simulink model "Task1"  (R2016a)
settings: Solver=VariableStepAuto  StartTime=0.0  StopTime=10.0  RelTol=1e-3
settings Model: Creator=Thomas  LastModifiedBy=Thomas

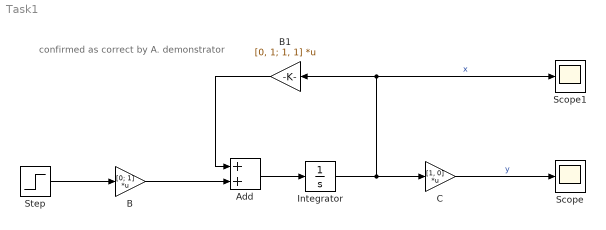
== system Task1 ==
  note: confirmed as correct by A. demonstrator
  Add : Sum
  B : Gain  Gain=[0; 1]  Multiplication=Matrix(K*u)
  B1 : Gain  Gain=[0, 1; 1, 1]  Multiplication=Matrix(K*u)
  C : Gain  Gain=[1, 0]  Multiplication=Matrix(K*u)
  Integrator : Integrator  InitialCondition=[1;1]
  Scope : Scope
  Scope1 : Scope
  Step : Step  SampleTime=0
  wires:
  Add/1 -> Integrator/1
  B1/1 -> Add/1
  Step/1 -> B/1
  B/1 -> Add/2
  Integrator/1 -> B1/1, Scope1/1, C/1  "x"
  C/1 -> Scope/1  "y"
